simulink model "top_model"  (R2018b)
settings: configuration reference "Config_Eng" (kept outside this file)
undefined symbols (not defined in the file or in its folder): HEVCtrl_Engine_torque_request, HEVCtrl_IdleStop_preparation_request, HEVCtrl_IdleStop_request, HEVCtrl_IdleStop_status
libraries: simulink x1, SignalEditorBlockLib x1
settings Model: DataDictionary=top_model.sldd  Creator=The MathWorks, Inc.  LastModifiedBy=m101062

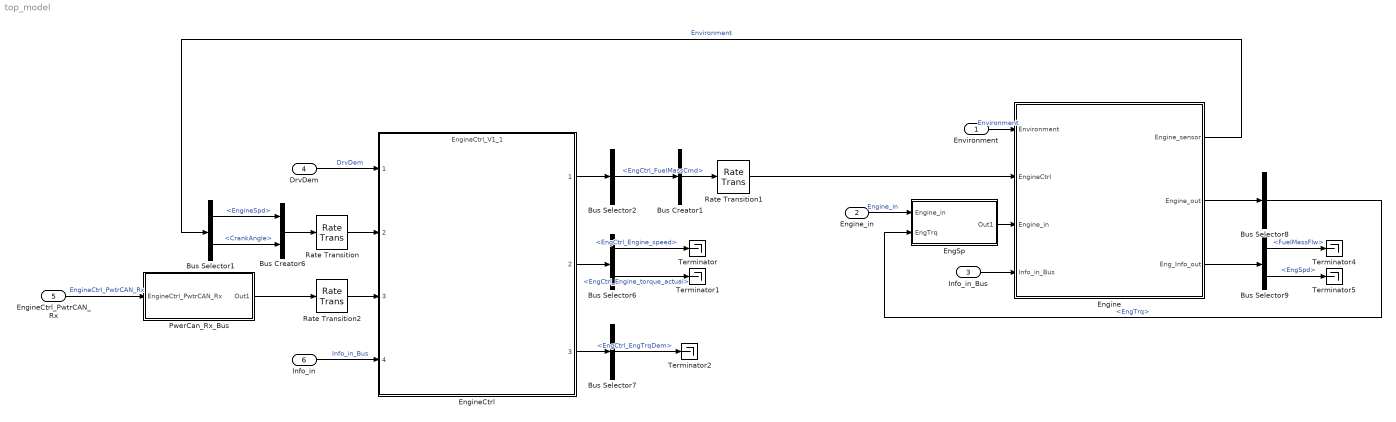
== system top_model ==
  Environment : Inport  OutDataTypeStr=Bus: Environment_Bus
      settings: AttributesFormatString=%<OutDataTypeStr>
  Engine_in : Inport  Port=2  OutDataTypeStr=Bus: Engine_in_Bus
      settings: AttributesFormatString=%<OutDataTypeStr>
  Info_in_Bus : Inport  Port=3  OutDataTypeStr=Bus: Eng_Info_in_Bus
      settings: AttributesFormatString=%<OutDataTypeStr>
  DrvDem : Inport  Port=4  OutDataTypeStr=Bus: Driver_demand_Bus
      settings: AttributesFormatString=%<OutDataTypeStr>
  EngineCtrl_PwtrCAN_Rx : Inport  Port=5  OutDataTypeStr=Bus: EngineCtrl_PwtrCAN_Rx_Bus
      settings: AttributesFormatString=<%<OutDataTypeStr>>
  Info_in : Inport  Port=6  OutDataTypeStr=Bus: EngineCtrl_Info_in_Bus
      settings: AttributesFormatString=%<OutDataTypeStr>
  Bus Creator1 : BusCreator  Inputs=1
  Bus Creator6 : BusCreator  Inputs=2
  Bus Selector1 : BusSelector  OutputSignals=EngineSpd,CrankAngle
  Bus Selector2 : BusSelector  OutputSignals=EngCtrl_FuelMassCmd
  Bus Selector6 : BusSelector  OutputSignals=EngCtrl_Engine_speed,EngCtrl_Engine_torque_actual
  Bus Selector7 : BusSelector  OutputSignals=EngCtrl_EngTrqDem
  Bus Selector8 : BusSelector  OutputSignals=EngTrq
  Bus Selector9 : BusSelector  OutputSignals=FuelMassFlw,EngSpd
  EngSp : Subsystem
  Engine : Subsystem  Variant=on
  EngineCtrl : ModelReference  ModelNameDialog=EngineCtrl_V1_1.slx  SimulationMode=Normal  ModelReferenceVersion=1.0.32
  PwerCan_Rx_Bus : Subsystem
  Rate Transition : RateTransition
  Rate Transition1 : RateTransition
  Rate Transition2 : RateTransition
  Terminator{,1..2,4..5} (5 alike) : Terminator
  wires:
  Info_in_Bus/1 -> Engine/4(Info_in_Bus)
  EngineCtrl_PwtrCAN_Rx/1 -> PwerCan_Rx_Bus/1(EngineCtrl_PwtrCAN_Rx)  "EngineCtrl_PwtrCAN_Rx"
  EngineCtrl/2 -> Bus Selector6/1
  EngineCtrl/3 -> Bus Selector7/1
  Engine/2(Engine_out) -> Bus Selector8/1
  Engine/3(Eng_Info_out) -> Bus Selector9/1
  Bus Selector6/1 -> Terminator/1  "<EngCtrl_Engine_speed>"
  Bus Selector6/2 -> Terminator1/1  "<EngCtrl_Engine_torque_actual>"
  Bus Selector7/1 -> Terminator2/1  "<EngCtrl_EngTrqDem>"
  Bus Selector9/1 -> Terminator4/1  "<FuelMassFlw>"
  Bus Selector9/2 -> Terminator5/1  "<EngSpd>"
  Engine/1(Engine_sensor) -> Bus Selector1/1  "Environment"
  Bus Selector1/2 -> Bus Creator6/2  "<CrankAngle>"
  Bus Selector1/1 -> Bus Creator6/1  "<EngineSpd>"
  Bus Creator6/1 -> Rate Transition/1
  Environment/1 -> Engine/1(Environment)  "Environment"
  Engine_in/1 -> EngSp/1(Engine_in)  "Engine_in"
  EngSp/1(Out1) -> Engine/3(Engine_in)
  Info_in/1 -> EngineCtrl/4  "Info_in_Bus"
  EngineCtrl/1 -> Bus Selector2/1
  Bus Creator1/1 -> Rate Transition1/1
  Bus Selector2/1 -> Bus Creator1/1  "<EngCtrl_FuelMassCmd>"
  DrvDem/1 -> EngineCtrl/1  "DrvDem"
  PwerCan_Rx_Bus/1(Out1) -> Rate Transition2/1
  Bus Selector8/1 -> EngSp/2(EngTrq)  "<EngTrq>"
  Rate Transition/1 -> EngineCtrl/2
  Rate Transition1/1 -> Engine/2(EngineCtrl)
  Rate Transition2/1 -> EngineCtrl/3

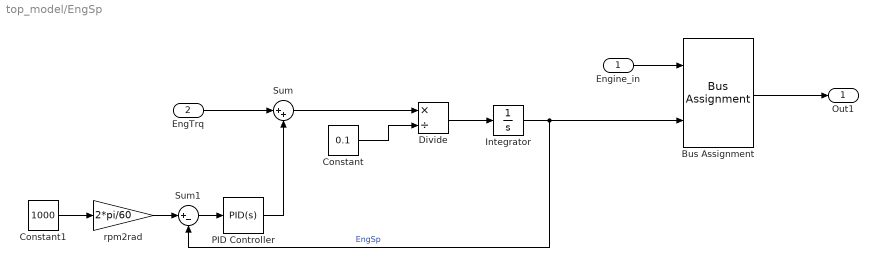
== system top_model/EngSp ==
  Engine_in : Inport
  EngTrq : Inport  Port=2
  Bus Assignment : BusAssignment  AssignedSignals=EngSpd
  Constant : Constant  Value=0.1
  Constant1 : Constant  Value=1000
  Divide : Product  Inputs=*/
  Integrator : Integrator  InitialCondition=100
  PID Controller : simulink/Continuous/PID Controller  Controller=PID  Form=Parallel  TimeDomain=Continuous-time  SampleTime=-1  IntegratorMethod=Forward Euler  FilterMethod=Forward Euler  ControllerParametersSource=internal  P=100  I=1000  D=0  UseFilter=on  N=100  TunerSelectOption=Transfer Function Based (PID Tuner App)  InitialConditionSource=internal  InitialConditionForIntegrator=0  InitialConditionForFilter=0  DifferentiatorICPrevScaledInput=0  ExternalReset=none  TrackingMode=off  Kt=1  LimitOutput=off  UpperSaturationLimit=inf  LowerSaturationLimit=-inf  LinearizeAsGain=on  AntiWindupMode=none  Kb=1  POutMin=[]  POutMax=[]  IOutMin=[]  IOutMax=[]  DOutMin=[]  DOutMax=[]  NOutMin=[]  NOutMax=[]  SumOutMin=[]  SumOutMax=[]  SaturationOutMin=[]  SaturationOutMax=[]  PParamMin=[]  PParamMax=[]  IParamMin=[]  IParamMax=[]  DParamMin=[]  DParamMax=[]  NParamMin=[]  NParamMax=[]  KbParamMin=[]  KbParamMax=[]  KtParamMin=[]  KtParamMax=[]  KbOutMin=[]  KbOutMax=[]  KtOutMin=[]  KtOutMax=[]  IntegratorOutMin=[]  IntegratorOutMax=[]  FilterOutMin=[]  FilterOutMax=[]  SumI1OutMin=[]  SumI1OutMax=[]  SumI2OutMin=[]  SumI2OutMax=[]  SumI3OutMin=[]  SumI3OutMax=[]  SumI4OutMin=[]  SumI4OutMax=[]  SumDOutMin=[]  SumDOutMax=[]  DifferentiatorOutMin=[]  DifferentiatorOutMax=[]  FilterDiffOutCoefMin=[]  FilterDiffOutCoefMax=[]  ReciprocalOutMin=[]  ReciprocalOutMax=[]  SumDenOutMin=[]  SumDenOutMax=[]  SumNumOutMin=[]  SumNumOutMax=[]  DivideOutMin=[]  DivideOutMax=[]  IntegratorContinuousStateAttributes=''  IntegratorStateMustResolveToSignalObject=off  IntegratorRTWStateStorageClass=Auto  FilterContinuousStateAttributes=''  FilterStateMustResolveToSignalObject=off  FilterRTWStateStorageClass=Auto  ParallelPVariant=InternalParameters  IdealPVariant=Disabled  IVariant=InternalParameters  DVariant=InternalParameters  IntegratorVariant=Continuous  SatVariant=Disabled  AWVariant=Passthrough  PCopyVariant=Disabled  TRVariant=Disabled  FdbkBlocksVariant=Forward  IdealPFdbkVariant=Disabled  SatFdbkVariant=Disabled  DerivativeFilterVariant=ContFilter  NVariant=InternalParameters  NCopyVariant=Disabled  FilterICVariant=InternalICsFilter  IntegratorICVariant=InternalICs  ExternalResetVariant=Disabled  TRSumVariant=Passthrough  SumFdbkVariant=Disabled  SumVariant=Sum_PID
  Sum : Sum  Inputs=|++
  Sum1 : Sum  Inputs=|+-
  rpm2rad : Gain  Gain=2*pi/60
  Out1 : Outport
  wires:
  Bus Assignment/1 -> Out1/1
  Engine_in/1 -> Bus Assignment/1
  Constant/1 -> Divide/2
  Constant1/1 -> rpm2rad/1
  PID Controller/1 -> Sum/2
  Sum1/1 -> PID Controller/1
  rpm2rad/1 -> Sum1/1
  Sum/1 -> Divide/1
  Integrator/1 -> Bus Assignment/2, Sum1/2  "EngSp"
  Divide/1 -> Integrator/1
  EngTrq/1 -> Sum/1

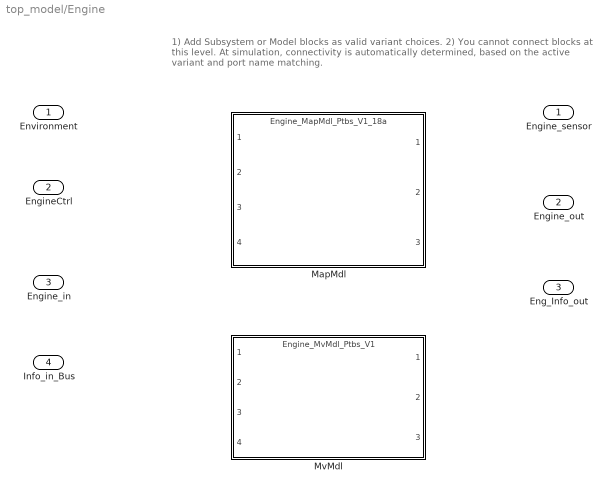
== system top_model/Engine ==
  note: 1) Add Subsystem or Model blocks as valid variant choices.
      | 2) You cannot connect blocks at this level. At simulation, connectivity is automatically
      | determined, based on the active variant and port name matching.
  Environment : Inport  OutDataTypeStr=Bus: Environment_Bus
      settings: AttributesFormatString=%<OutDataTypeStr>
  EngineCtrl : Inport  Port=2  OutDataTypeStr=Bus: EngineCtrl_Bus
      settings: AttributesFormatString=%<OutDataTypeStr>
  Engine_in : Inport  Port=3  OutDataTypeStr=Bus: Engine_in_Bus
      settings: AttributesFormatString=%<OutDataTypeStr>
  Info_in_Bus : Inport  Port=4  OutDataTypeStr=Bus: Eng_Info_in_Bus
      settings: AttributesFormatString=%<OutDataTypeStr>
  MapMdl : ModelReference  DisableCoverage=on  ModelNameDialog=Engine_MapMdl_Ptbs_V1_18a.slx  VariantControl=VarObj_Eng_MapMdl  ModelReferenceVersion=1.1341
  MvMdl : ModelReference  ModelNameDialog=Engine_MvMdl_Ptbs_V1.slx  VariantControl=VarObj_Eng_MvMdl  ModelReferenceVersion=1.1331
  Engine_sensor : Outport  OutDataTypeStr=Bus: Engine_sensor_Bus
      settings: AttributesFormatString=%<OutDataTypeStr>
  Engine_out : Outport  Port=2  OutDataTypeStr=Bus: Engine_out_Bus
      settings: AttributesFormatString=%<OutDataTypeStr>
  Eng_Info_out : Outport  Port=3  OutDataTypeStr=Bus: Eng_Info_out_Bus
      settings: AttributesFormatString=%<OutDataTypeStr>

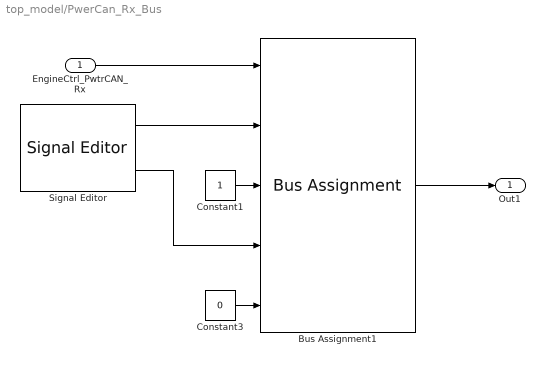
== system top_model/PwerCan_Rx_Bus ==
  EngineCtrl_PwtrCAN_Rx : Inport
  Bus Assignment1 : BusAssignment  AssignedSignals=HEVCtrl_Engine_torque_request,HEVCtrl_IdleStop_preparation_request,HEVCtrl_IdleStop_request,HEVCtrl_IdleStop_status
  Constant1 : Constant  OutDataTypeStr=Inherit: Inherit via back propagation
  Constant3 : Constant  Value=0
  Signal Editor : SignalEditorBlockLib/Signal Editor  FileName=TestSignal.mat  ActiveScenario=Scenario  ActiveSignal=IdleStop_request  IsBus=off  OutputBusObjectStr=Bus: BusObject  SampleTime=0  Interpolate=off  ZeroCross=off  OutputAfterFinalValue=Setting to zero  Unit=inherit
  Out1 : Outport
  wires:
  Bus Assignment1/1 -> Out1/1
  EngineCtrl_PwtrCAN_Rx/1 -> Bus Assignment1/1
  Signal Editor/1 -> Bus Assignment1/2
  Constant1/1 -> Bus Assignment1/3
  Signal Editor/2 -> Bus Assignment1/4
  Constant3/1 -> Bus Assignment1/5
